simulink model "smartCart5_1work"  (R2016a)
settings: Solver=FixedStepDiscrete  StartTime=0.0  StopTime=inf  FixedStep=1  RelTol=1e-3
libraries: simulink x213, hdlsllib x84
(part 2 of 4)

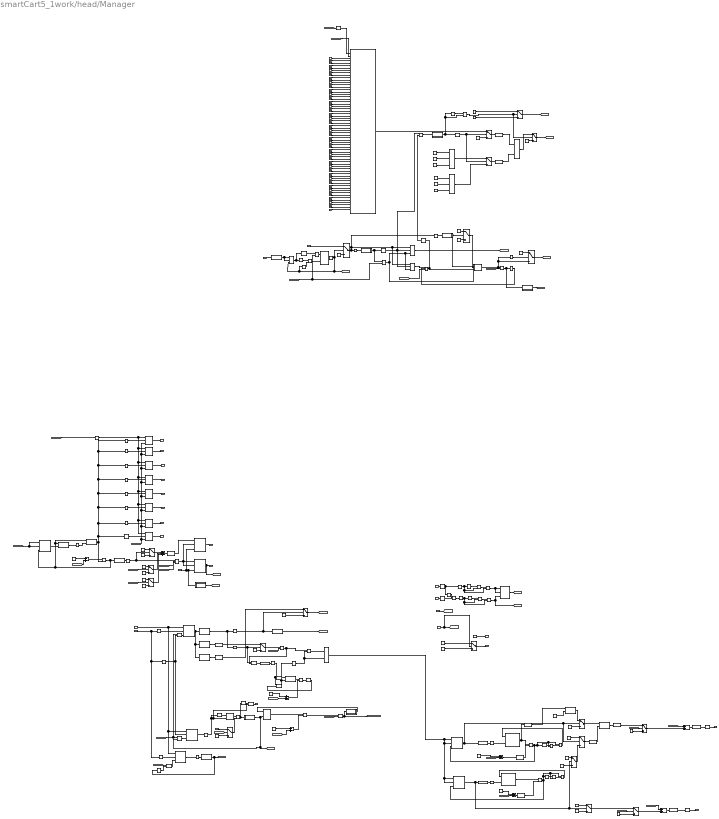
== system smartCart5_1work/head/Manager ==
  note: Декодер команд
  note: Схема декодирования команд
  note: Схема синхр
  note: Схема включения и выключения
  note: Схема управления приёмника
  note: Схема управления передатчиком
  AdrrIN : Inport  OutDataTypeStr=uint8
  DataIN : Inport  Port=2  OutDataTypeStr=uint32
  Start : Inport  Port=3  OutDataTypeStr=boolean
  Stop : Inport  Port=4  OutDataTypeStr=boolean
  RD : Inport  Port=5  OutDataTypeStr=boolean
  STEP : Inport  Port=6  OutDataTypeStr=uint8
  RST_IRQ : Inport  Port=7  OutDataTypeStr=boolean
  Number_write_byte : Inport  Port=8  OutDataTypeStr=uint8
  ON_TRANSMITE : Inport  Port=9  OutDataTypeStr=boolean
  time_pause : Inport  Port=10  OutDataTypeStr=uint32
  data_in_0 : Inport  Port=11  OutDataTypeStr=uint32
  data_in_1 : Inport  Port=12  OutDataTypeStr=uint32
  data_in_2 : Inport  Port=13  OutDataTypeStr=uint32
  data_in_3 : Inport  Port=14  OutDataTypeStr=uint32
  data_in_4 : Inport  Port=15  OutDataTypeStr=uint32
  data_in_5 : Inport  Port=16  OutDataTypeStr=uint32
  data_in_6 : Inport  Port=17  OutDataTypeStr=uint32
  data_in_7 : Inport  Port=18  OutDataTypeStr=uint32
  data_in_8 : Inport  Port=19  OutDataTypeStr=uint32
  data_in_9 : Inport  Port=20  OutDataTypeStr=uint32
  data_in_10 : Inport  Port=21  OutDataTypeStr=uint32
  data_in_11 : Inport  Port=22  OutDataTypeStr=uint32
  data_in_12 : Inport  Port=23  OutDataTypeStr=uint32
  data_in_13 : Inport  Port=24  OutDataTypeStr=uint32
  data_in_14 : Inport  Port=25  OutDataTypeStr=uint32
  data_in_15 : Inport  Port=26  OutDataTypeStr=uint32
  data_in_16 : Inport  Port=27  OutDataTypeStr=uint32
  data_in_17 : Inport  Port=28  OutDataTypeStr=uint32
  data_in_18 : Inport  Port=29  OutDataTypeStr=uint32
  data_in_19 : Inport  Port=30  OutDataTypeStr=uint32
  data_in_20 : Inport  Port=31  OutDataTypeStr=uint32
  data_in_21 : Inport  Port=32  OutDataTypeStr=uint32
  data_in_22 : Inport  Port=33  OutDataTypeStr=uint32
  data_in_23 : Inport  Port=34  OutDataTypeStr=uint32
  data_in_24 : Inport  Port=35  OutDataTypeStr=uint32
  data_in_25 : Inport  Port=36  OutDataTypeStr=uint32
  data_in_26 : Inport  Port=37  OutDataTypeStr=uint32
  data_in_27 : Inport  Port=38  OutDataTypeStr=uint32
  data_in_28 : Inport  Port=39  OutDataTypeStr=uint32
  data_in_29 : Inport  Port=40  OutDataTypeStr=uint32
  data_in_30 : Inport  Port=41  OutDataTypeStr=uint32
  data_in_31 : Inport  Port=42  OutDataTypeStr=uint32
  data_in_32 : Inport  Port=43  OutDataTypeStr=uint32
  data_in_33 : Inport  Port=44  OutDataTypeStr=uint32
  data_in_34 : Inport  Port=45  OutDataTypeStr=uint32
  data_in_35 : Inport  Port=46  OutDataTypeStr=uint32
  data_in_36 : Inport  Port=47  OutDataTypeStr=uint32
  data_in_37 : Inport  Port=48  OutDataTypeStr=uint32
  data_in_38 : Inport  Port=49  OutDataTypeStr=uint32
  data_in_39 : Inport  Port=50  OutDataTypeStr=uint32
  data_in_40 : Inport  Port=51  OutDataTypeStr=uint32
  data_in_41 : Inport  Port=52  OutDataTypeStr=uint32
  data_in_42 : Inport  Port=53  OutDataTypeStr=uint32
  data_in_43 : Inport  Port=54  OutDataTypeStr=uint32
  data_in_44 : Inport  Port=55  OutDataTypeStr=uint32
  data_in_45 : Inport  Port=56  OutDataTypeStr=uint32
  data_in_46 : Inport  Port=57  OutDataTypeStr=uint32
  data_in_47 : Inport  Port=58  OutDataTypeStr=uint32
  data_in_48 : Inport  Port=59  OutDataTypeStr=uint32
  data_in_49 : Inport  Port=60  OutDataTypeStr=uint32
  data_in_50 : Inport  Port=61  OutDataTypeStr=uint32
  data_in_51 : Inport  Port=62  OutDataTypeStr=uint32
  data_in_52 : Inport  Port=63  OutDataTypeStr=uint32
  data_in_53 : Inport  Port=64  OutDataTypeStr=uint32
  data_in_54 : Inport  Port=65  OutDataTypeStr=uint32
  data_in_55 : Inport  Port=66  OutDataTypeStr=uint32
  data_in_56 : Inport  Port=67  OutDataTypeStr=uint32
  data_in_57 : Inport  Port=68  OutDataTypeStr=uint32
  data_in_58 : Inport  Port=69  OutDataTypeStr=uint32
  data_in_59 : Inport  Port=70  OutDataTypeStr=uint32
  data_in_60 : Inport  Port=71  OutDataTypeStr=uint32
  data_in_61 : Inport  Port=72  OutDataTypeStr=uint32
  data_in_62 : Inport  Port=73  OutDataTypeStr=uint32
  data_in_63 : Inport  Port=74  OutDataTypeStr=uint32
  Add{,1..5,7} (7 alike) : Sum
  Add6 : Sum  Inputs=+++
  Atomic Subsystem : Subsystem  TreatAsAtomicUnit=on
  Bit Concat : hdlsllib/HDL Operations/Bit Concat  numInputs=2
  Bit Concat1 : hdlsllib/HDL Operations/Bit Concat  numInputs=2
  Bit Concat2 : hdlsllib/HDL Operations/Bit Concat  numInputs=3
  Bit Concat3 : hdlsllib/HDL Operations/Bit Concat  numInputs=3
  Bit Concat4 : hdlsllib/HDL Operations/Bit Concat  numInputs=2
  Bit Slice3 : hdlsllib/HDL Operations/Bit Slice  lidx=1  ridx=0
  Bit Slice4 : hdlsllib/HDL Operations/Bit Slice  lidx=9  ridx=2
  Bit Slice5 : hdlsllib/HDL Operations/Bit Slice  lidx=17  ridx=10
  Compare To Constant{,1..6,10,12,22,26} (11 alike) : simulink/Logic and Bit Operations/Compare To Constant  relop===  const=1  OutDataTypeStr=boolean
  Compare To Constant11 : simulink/Logic and Bit Operations/Compare To Constant  relop===  const=4  OutDataTypeStr=boolean
  Compare To Constant13 : simulink/Logic and Bit Operations/Compare To Constant  relop===  const=2  OutDataTypeStr=boolean
  Compare To Constant14 : simulink/Logic and Bit Operations/Compare To Constant  relop===  const=5  OutDataTypeStr=boolean
  Compare To Constant15 : simulink/Logic and Bit Operations/Compare To Constant  relop===  const=6  OutDataTypeStr=boolean
  Compare To Constant16 : simulink/Logic and Bit Operations/Compare To Constant  relop===  const=7  OutDataTypeStr=boolean
  Compare To Constant17 : simulink/Logic and Bit Operations/Compare To Constant  relop===  const=8  OutDataTypeStr=boolean
  Compare To Constant18 : simulink/Logic and Bit Operations/Compare To Constant  relop=~=  const=255  OutDataTypeStr=boolean
  Compare To Constant19 : simulink/Logic and Bit Operations/Compare To Constant  relop===  const=100  OutDataTypeStr=boolean
  Compare To Constant23 : simulink/Logic and Bit Operations/Compare To Constant  relop===  const=255  OutDataTypeStr=boolean
  Compare To Constant24 : simulink/Logic and Bit Operations/Compare To Constant  relop===  const=0  OutDataTypeStr=boolean
  Compare To Constant25 : simulink/Logic and Bit Operations/Compare To Constant  relop===  const=6  OutDataTypeStr=boolean
  Compare To Constant7 : simulink/Logic and Bit Operations/Compare To Constant  relop===  const=2  OutDataTypeStr=boolean
  Compare To Constant8 : simulink/Logic and Bit Operations/Compare To Constant  relop===  const=3  OutDataTypeStr=boolean
  Compare To Constant9 : simulink/Logic and Bit Operations/Compare To Constant  relop===  const=2  OutDataTypeStr=boolean
  Constant{,2,12..15,23,25,28,36} (10 alike) : Constant  Value=0  OutDataTypeStr=uint8  SampleTime=-1
  Constant{1,3,7,10,24} (5 alike) : Constant  OutDataTypeStr=uint8  SampleTime=-1
  Constant11 : Constant  Value=4  OutDataTypeStr=uint8  SampleTime=-1
  Constant{5,16,18,26} (4 alike) : Constant  OutDataTypeStr=boolean  SampleTime=-1
  Constant{6,17,22,31,33..34,38} (7 alike) : Constant  Value=0  OutDataTypeStr=uint32  SampleTime=-1
  Constant19 : Constant  Value=0  OutDataTypeStr=boolean  SampleTime=-1
  Constant20 : Constant  Value=0  OutDataTypeStr=boolean  SampleTime=-1
  Constant21 : Constant  Value=0  OutDataTypeStr=boolean  SampleTime=-1
  Constant27 : Constant  Value=2  OutDataTypeStr=uint8  SampleTime=-1
  Constant29 : Constant  Value=255  OutDataTypeStr=uint8  SampleTime=-1
  Constant30 : Constant  OutDataTypeStr=uint32  SampleTime=-1
  Constant32 : Constant  Value=2  OutDataTypeStr=uint32  SampleTime=-1
  Constant35 : Constant  Value=255  OutDataTypeStr=uint8  SampleTime=-1
  Constant37 : Constant  Value=3  OutDataTypeStr=uint32  SampleTime=-1
  Constant4 : Constant  Value=2  OutDataTypeStr=uint8  SampleTime=-1
  Constant40 : Constant  OutDataTypeStr=uint32  SampleTime=-1
  Constant8 : Constant  OutDataTypeStr=uint32  SampleTime=-1
  Constant9 : Constant  Value=2  OutDataTypeStr=uint8  SampleTime=-1
  Data Type Conversion{,3..4,7..8} (5 alike) : DataTypeConversion  OutDataTypeStr=uint8
  Data Type Conversion1 : DataTypeConversion  OutDataTypeStr=uint32
  Data Type Conversion10 : DataTypeConversion  OutDataTypeStr=fixdt(0,2,0)
  Data Type Conversion11 : DataTypeConversion  OutDataTypeStr=fixdt(0,3,0)
  Data Type Conversion12 : DataTypeConversion  OutDataTypeStr=uint32
  Data Type Conversion5 : DataTypeConversion  OutDataTypeStr=uint32
  Data Type Conversion6 : DataTypeConversion  OutDataTypeStr=fixdt(0,4,0)
  Data Type Conversion9 : DataTypeConversion  OutDataTypeStr=fixdt(0,4,0)
  Delay{,1..3,5..17} (17 alike) : Delay  DelayLength=1  InitialCondition=0
  Delay4 : Delay  DelayLength=3  InitialCondition=0
  HDL Counter1 : hdlsllib/HDL Operations/HDL Counter  CountType=Free running  CountInit=0  CountStep=1  CountMax=25  CountFromType=Initial value  CountFrom=0  CountResetPort=on  CountLoadPort=off  CountEnbPort=on  CountDirPort=off  CountDataType=Unsigned  CountWordLen=4  CountFracLen=0  CountSampTime=1
  HDL Counter10 : hdlsllib/HDL Operations/HDL Counter  CountType=Free running  CountInit=255  CountStep=1  CountMax=25  CountFromType=Initial value  CountFrom=255  CountResetPort=on  CountLoadPort=off  CountEnbPort=on  CountDirPort=off  CountDataType=Unsigned  CountWordLen=8  CountFracLen=0  CountSampTime=1
  HDL Counter12 : hdlsllib/HDL Operations/HDL Counter  CountType=Count limited  CountInit=0  CountStep=1  CountMax=100  CountFromType=Initial value  CountFrom=0  CountResetPort=on  CountLoadPort=off  CountEnbPort=on  CountDirPort=off  CountDataType=Unsigned  CountWordLen=8  CountFracLen=0  CountSampTime=1
  HDL Counter13 : hdlsllib/HDL Operations/HDL Counter  CountType=Free running  CountInit=0  CountStep=1  CountMax=5208*2  CountFromType=Initial value  CountFrom=0  CountResetPort=on  CountLoadPort=off  CountEnbPort=on  CountDirPort=off  CountDataType=Unsigned  CountWordLen=32  CountFracLen=0  CountSampTime=1
  HDL Counter2 : hdlsllib/HDL Operations/HDL Counter  CountType=Free running  CountInit=0  CountStep=1  CountMax=25  CountFromType=Initial value  CountFrom=0  CountResetPort=on  CountLoadPort=off  CountEnbPort=on  CountDirPort=off  CountDataType=Unsigned  CountWordLen=4  CountFracLen=0  CountSampTime=1
  HDL Counter3 : hdlsllib/HDL Operations/HDL Counter  CountType=Free running  CountInit=0  CountStep=1  CountMax=25  CountFromType=Initial value  CountFrom=0  CountResetPort=on  CountLoadPort=off  CountEnbPort=on  CountDirPort=off  CountDataType=Unsigned  CountWordLen=8  CountFracLen=0  CountSampTime=1
  HDL Counter4 : hdlsllib/HDL Operations/HDL Counter  CountType=Free running  CountInit=0  CountStep=1  CountMax=25  CountFromType=Initial value  CountFrom=0  CountResetPort=on  CountLoadPort=off  CountEnbPort=on  CountDirPort=off  CountDataType=Unsigned  CountWordLen=4  CountFracLen=0  CountSampTime=1
  HDL Counter5 : hdlsllib/HDL Operations/HDL Counter  CountType=Free running  CountInit=0  CountStep=1  CountMax=25  CountFromType=Initial value  CountFrom=0  CountResetPort=off  CountLoadPort=off  CountEnbPort=on  CountDirPort=off  CountDataType=Unsigned  CountWordLen=1  CountFracLen=0  CountSampTime=1
  HDL Counter6 : hdlsllib/HDL Operations/HDL Counter  CountType=Free running  CountInit=0  CountStep=1  CountMax=25  CountFromType=Initial value  CountFrom=0  CountResetPort=off  CountLoadPort=off  CountEnbPort=on  CountDirPort=off  CountDataType=Unsigned  CountWordLen=1  CountFracLen=0  CountSampTime=1
  HDL Counter7 : hdlsllib/HDL Operations/HDL Counter  CountType=Free running  CountInit=0  CountStep=1  CountMax=25  CountFromType=Initial value  CountFrom=0  CountResetPort=off  CountLoadPort=off  CountEnbPort=on  CountDirPort=off  CountDataType=Unsigned  CountWordLen=1  CountFracLen=0  CountSampTime=1
  HDL Counter8 : hdlsllib/HDL Operations/HDL Counter  CountType=Free running  CountInit=0  CountStep=1  CountMax=25  CountFromType=Initial value  CountFrom=0  CountResetPort=on  CountLoadPort=off  CountEnbPort=on  CountDirPort=off  CountDataType=Unsigned  CountWordLen=1  CountFracLen=0  CountSampTime=1
  HDL Counter9 : hdlsllib/HDL Operations/HDL Counter  CountType=Free running  CountInit=0  CountStep=1  CountMax=25  CountFromType=Initial value  CountFrom=0  CountResetPort=on  CountLoadPort=on  CountEnbPort=on  CountDirPort=off  CountDataType=Unsigned  CountWordLen=8  CountFracLen=0  CountSampTime=1
  Logical Operator{,2,7,10} (4 alike) : Logic  Operator=XOR  AllPortsSameDT=off  OutDataTypeStr=boolean
  Logical Operator{1,3..4,6,8..9,12,15,17,19,26,32} (12 alike) : Logic  AllPortsSameDT=off  OutDataTypeStr=boolean
  Logical Operator{5,11,16,18,25,31} (6 alike) : Logic  Operator=NOT  AllPortsSameDT=off  OutDataTypeStr=boolean
  Logical Operator{13..14,20,22,24,28,30} (7 alike) : Logic  Operator=OR  AllPortsSameDT=off  OutDataTypeStr=boolean
  Logical Operator23 : Logic  Operator=OR  Inputs=3  AllPortsSameDT=off  OutDataTypeStr=boolean
  Logical Operator27 : Logic  Inputs=3  AllPortsSameDT=off  OutDataTypeStr=boolean
  Logical Operator29 : Logic  Operator=NOT  Inputs=3  AllPortsSameDT=off  OutDataTypeStr=boolean
  Relational Operator{,1..4,6..8} (8 alike) : RelationalOperator  Operator===  OutDataTypeStr=boolean
  Switch{1..19,21} (20 alike) : Switch  Criteria=u2 ~= 0
  Unit Delay Enabled Resettable{,1..2,5..13,15,25} (14 alike) : simulink/Additional Math & Discrete/Additional Discrete/Unit Delay Enabled Resettable  vinit=0.0  tsamp=-1
  Unit Delay Enabled Resettable{3..4,14,16,26,28} (6 alike) : simulink/Additional Math & Discrete/Additional Discrete/Unit Delay Enabled Resettable  vinit=0  tsamp=-1
  signal_edg : Subsystem  TreatAsAtomicUnit=on
  signal_edg1 : Subsystem  TreatAsAtomicUnit=on
  signal_edg10 : Subsystem  TreatAsAtomicUnit=on
  signal_edg11 : Subsystem  TreatAsAtomicUnit=on
  signal_edg12 : Subsystem  TreatAsAtomicUnit=on
  signal_edg2 : Subsystem  TreatAsAtomicUnit=on
  signal_edg3 : Subsystem  TreatAsAtomicUnit=on
  signal_edg4 : Subsystem  TreatAsAtomicUnit=on
  signal_edg6 : Subsystem  TreatAsAtomicUnit=on
  signal_edg7 : Subsystem  TreatAsAtomicUnit=on
  signal_edg8 : Subsystem  TreatAsAtomicUnit=on
  signal_edg9 : Subsystem  TreatAsAtomicUnit=on
  addrout : Outport  OutDataTypeStr=uint8
  DATA_OUT : Outport  Port=2  OutDataTypeStr=uint32
  Out1 : Outport  Port=3  OutDataTypeStr=uint8
  Out2 : Outport  Port=4  OutDataTypeStr=uint8
  Out3 : Outport  Port=5  OutDataTypeStr=uint8
  Out4 : Outport  Port=6  OutDataTypeStr=uint8
  Out5 : Outport  Port=7  OutDataTypeStr=uint8
  Out6 : Outport  Port=8  OutDataTypeStr=uint8
  Out7 : Outport  Port=9  OutDataTypeStr=uint8
  Out8 : Outport  Port=10  OutDataTypeStr=uint8
  irq : Outport  Port=11  OutDataTypeStr=boolean
  addr_mux : Outport  Port=12  OutDataTypeStr=uint8
  data_mux : Outport  Port=13  OutDataTypeStr=uint32
  STATUS : Outport  Port=14  OutDataTypeStr=uint32
  rd_switch : Outport  Port=15  OutDataTypeStr=boolean
  wires:
  Compare To Constant/1 -> Logical Operator1/2, Logical Operator/2, Delay/1
  Delay/1 -> Logical Operator/1
  Logical Operator/1 -> Logical Operator1/1
  Logical Operator1/1 -> Unit Delay Enabled Resettable/2, Unit Delay Enabled Resettable/1
  Compare To Constant1/1 -> Logical Operator3/2, Logical Operator2/2, Delay1/1
  Delay1/1 -> Logical Operator2/1
  Logical Operator2/1 -> Logical Operator3/1
  Logical Operator5/1 -> Logical Operator4/1
  Logical Operator4/1 -> Compare To Constant1/1
  Logical Operator3/1 -> Unit Delay Enabled Resettable/3, [RST]
  Unit Delay Enabled Resettable/1 -> [EN]
  HDL Counter2/1 -> Relational Operator2/1
  Bit Slice4/1 -> Data Type Conversion7/1
  Bit Slice5/1 -> Data Type Conversion8/1
  Bit Slice3/1 -> Compare To Constant10/1, Compare To Constant9/1
  Data Type Conversion8/1 -> Switch9/1
  Constant14/1 -> Switch9/3
  Data Type Conversion7/1 -> Switch10/1
  Constant15/1 -> Switch10/3
  Unit Delay Enabled Resettable1/1 -> Bit Slice5/1, Bit Slice4/1, Bit Slice3/1
  AdrrIN/1 -> Compare To Constant25/1, Compare To Constant13/1, Compare To Constant12/1
  Compare To Constant12/1 -> Unit Delay Enabled Resettable1/2
  HDL Counter1/1 -> Relational Operator1/1, Data Type Conversion/1
  Constant1/1 -> Switch1/1
  Constant2/1 -> Switch1/3
  Switch2/1 -> Bit Concat/1
  Constant/1 -> Switch2/3
  Constant4/1 -> Switch3/1
  Data Type Conversion/1 -> Bit Concat1/1
  Constant5/1 -> Bit Concat1/2
  Bit Concat1/1 -> Switch2/1
  Bit Concat/1 -> Data Type Conversion1/1
  Switch10/1 -> Relational Operator/1
  STEP/1 -> [INST_WORK_VAL]
  [INST_WORK_VAL] -> Relational Operator/2
  [INST_WORK_VAL] -> Add/2
  Constant9/1 -> Add/1
  Logical Operator8/1 -> Unit Delay Enabled Resettable4/2, Unit Delay Enabled Resettable4/1, Unit Delay Enabled Resettable3/2, Unit Delay Enabled Resettable3/1
  Data Type Conversion1/1 -> Switch12/1
  Constant22/1 -> Switch12/3
  [INST_WORK] -> Switch12/2
  Switch1/1 -> Switch13/1
  [INST_WORK] -> Switch13/2
  Constant23/1 -> Switch13/3
  Switch12/1 -> Add2/2
  Switch13/1 -> Add1/2
  Add1/1 -> Data Type Conversion4/1
  Add2/1 -> Data Type Conversion5/1
  Delay6/1 -> Logical Operator17/2, Logical Operator8/2
  Add/1 -> Data Type Conversion6/1
  Data Type Conversion6/1 -> Relational Operator2/2
  [INST_WORK_VAL] -> Add3/2
  Constant24/1 -> Add3/1
  Add3/1 -> Data Type Conversion9/1
  Data Type Conversion9/1 -> Relational Operator1/2
  Delay7/1 -> DATA_OUT/1
  Data Type Conversion5/1 -> Delay7/1
  Delay8/1 -> addrout/1
  Data Type Conversion4/1 -> Delay8/1
  Constant3/1 -> Switch14/1
  Switch3/1 -> Data Type Conversion10/1
  Data Type Conversion10/1 -> Bit Concat/2
  Switch14/1 -> Switch3/3
  Constant25/1 -> Switch14/3
  Logical Operator17/1 -> Logical Operator8/1
  Relational Operator/1 -> Logical Operator19/2, Logical Operator17/1
  Unit Delay Enabled Resettable3/1 -> HDL Counter6/1, Switch3/2, Switch2/2
  Unit Delay Enabled Resettable4/1 -> Switch14/2, Switch1/2, HDL Counter7/1
  [addr_wr] -> Add1/1
  [data_wr] -> Add2/1
  Logical Operator7/1 -> Logical Operator6/2
  Delay2/1 -> Logical Operator7/1
  Relational Operator1/1 -> Unit Delay Enabled Resettable3/3, Logical Operator6/1, Logical Operator7/2, Delay2/1
  Logical Operator6/1 -> HDL Counter1/1
  Logical Operator10/1 -> Logical Operator9/2
  Delay3/1 -> Logical Operator10/1
  Relational Operator2/1 -> Unit Delay Enabled Resettable4/3, Delay3/1, Logical Operator9/1, Logical Operator10/2
  Logical Operator9/1 -> HDL Counter2/1
  Compare To Constant10/1 -> Logical Operator19/1, Switch10/2
  Logical Operator11/1 -> HDL Counter4/1
  HDL Counter4/1 -> Relational Operator4/1
  [INST_WORK_VAL] -> Add5/2
  Add5/1 -> Relational Operator4/2
  Constant10/1 -> Add5/1
  Logical Operator12/1 -> Delay6/1, HDL Counter4/2
  Relational Operator4/1 -> Logical Operator18/1
  Logical Operator18/1 -> Logical Operator12/2
  HDL Counter5/1 -> Compare To Constant3/1
  Logical Operator19/1 -> HDL Counter5/1
  Compare To Constant3/1 -> Logical Operator12/1, Logical Operator11/1
  HDL Counter6/1 -> Compare To Constant4/1
  Compare To Constant4/1 -> HDL Counter1/2
  HDL Counter7/1 -> Compare To Constant5/1
  Compare To Constant5/1 -> HDL Counter2/2
  Compare To Constant9/1 -> Switch9/2, signal_edg/1(In1)
  Switch9/1 -> [RD_BYTE_VAL]
  RD/1 -> Switch5/2, [INST_WORK]
  Logical Operator13/1 -> Unit Delay Enabled Resettable2/3
  [RST] -> Logical Operator14/1, Logical Operator13/1
  Logical Operator14/1 -> Unit Delay Enabled Resettable1/3
  signal_edg/1(Out1) -> [RD_BYTE]
  [RD_BYTE] -> Unit Delay Enabled Resettable5/1, Unit Delay Enabled Resettable5/2
  Unit Delay Enabled Resettable5/1 -> HDL Counter8/2
  HDL Counter8/1 -> Compare To Constant2/1
  Compare To Constant2/1 -> HDL Counter3/2
  Constant7/1 -> Add4/1
  Add4/1 -> Relational Operator3/1
  [INST_WORK_VAL] -> Add4/2
  Relational Operator3/1 -> signal_edg4/1(In1), Unit Delay Enabled Resettable5/3, HDL Counter8/1, HDL Counter3/1
  Compare To Constant6/1 -> Unit Delay Enabled Resettable6/2
  Compare To Constant7/1 -> Unit Delay Enabled Resettable7/2
  Compare To Constant8/1 -> Unit Delay Enabled Resettable8/2
  Compare To Constant11/1 -> Unit Delay Enabled Resettable9/2
  Compare To Constant14/1 -> Unit Delay Enabled Resettable10/2
  Compare To Constant15/1 -> Unit Delay Enabled Resettable11/2
  Compare To Constant16/1 -> Unit Delay Enabled Resettable12/2
  Compare To Constant17/1 -> Unit Delay Enabled Resettable13/2
  HDL Counter3/1 -> Compare To Constant17/1, Compare To Constant16/1, Compare To Constant14/1, Compare To Constant11/1, Compare To Constant8/1, Compare To Constant6/1, Compare To Constant7/1, Compare To Constant15/1, Relational Operator3/2
  Unit Delay Enabled Resettable6/1 -> Out1/1
  Unit Delay Enabled Resettable7/1 -> Out2/1
  Unit Delay Enabled Resettable8/1 -> Out3/1
  Unit Delay Enabled Resettable9/1 -> Out4/1
  Unit Delay Enabled Resettable10/1 -> Out5/1
  Unit Delay Enabled Resettable11/1 -> Out6/1
  Unit Delay Enabled Resettable12/1 -> Out7/1
  Unit Delay Enabled Resettable13/1 -> Out8/1
  [RST] -> Unit Delay Enabled Resettable9/3, Unit Delay Enabled Resettable8/3, Unit Delay Enabled Resettable7/3, Unit Delay Enabled Resettable6/3, Unit Delay Enabled Resettable10/3, Unit Delay Enabled Resettable11/3, Unit Delay Enabled Resettable12/3, Unit Delay Enabled Resettable13/3
  Delay4/1 -> Unit Delay Enabled Resettable9/1, Unit Delay Enabled Resettable12/1, Unit Delay Enabled Resettable13/1, Unit Delay Enabled Resettable11/1, Unit Delay Enabled Resettable10/1, Unit Delay Enabled Resettable8/1, Unit Delay Enabled Resettable7/1, Unit Delay Enabled Resettable6/1
  Unit Delay Enabled Resettable14/1 -> [interrypt], irq/1
  RST_IRQ/1 -> Unit Delay Enabled Resettable26/3, signal_edg10/1(In1), Unit Delay Enabled Resettable14/3
  Constant6/1 -> Switch5/1
  Constant8/1 -> Switch5/3
  Switch5/1 -> data_mux/1
  Constant11/1 -> addr_mux/1
  [RD_BYTE_VAL] -> Delay4/1
  ? -> ?
  Atomic Subsystem/1(DataOut) -> Switch6/1
  Constant17/1 -> Switch6/3
  Constant16/1 -> Bit Concat2/3
  Constant18/1 -> Bit Concat2/2
  Constant19/1 -> Bit Concat2/1
  Constant20/1 -> Bit Concat3/3
  Constant21/1 -> Bit Concat3/2
  Constant26/1 -> Bit Concat3/1
  Bit Concat2/1 -> Switch7/1
  Bit Concat3/1 -> Switch7/3
  Switch6/1 -> Data Type Conversion3/1
  Switch7/1 -> Data Type Conversion11/1
  Data Type Conversion3/1 -> Bit Concat4/1
  Data Type Conversion11/1 -> Bit Concat4/2
  signal_edg2/1(Out1) -> Delay11/1, Logical Operator22/2, Delay10/1
  Delay10/1 -> Switch7/2, Switch6/2
  Delay11/1 -> Logical Operator22/1
  Logical Operator22/1 -> Switch16/2, Switch8/2
  Constant27/1 -> Switch8/1
  Constant28/1 -> Switch8/3
  Bit Concat4/1 -> Switch16/1
  [count_wr] -> Delay12/1
  Unit Delay Enabled Resettable26/1 -> STATUS/1
  Delay5/1 -> Switch11/2, Logical Operator23/1
  Logical Operator23/1 -> Unit Delay Enabled Resettable26/2, Unit Delay Enabled Resettable14/1, Unit Delay Enabled Resettable14/2
  Constant30/1 -> Switch11/1
  Constant31/1 -> Switch11/3
  Switch11/1 -> Add6/1
  Switch15/1 -> Add6/2
  Constant32/1 -> Switch15/1
  Constant33/1 -> Switch15/3
  [IRQ_TRANSMIT] -> Switch15/2
  [IRQ_TRANSMIT] -> Logical Operator23/2
  signal_edg4/1(Out1) -> Delay5/1
  Add6/1 -> Data Type Conversion12/1
  Data Type Conversion12/1 -> Unit Delay Enabled Resettable26/1
  HDL Counter10/1 -> Relational Operator7/1
  signal_edg12/1(Out1) -> Logical Operator13/2, [byte_done], HDL Counter10/2
  Start/1 -> Delay13/1
  Delay13/1 -> Logical Operator5/1, Compare To Constant/1
  Stop/1 -> Delay14/1
  Delay14/1 -> Logical Operator4/2
  Constant34/1 -> Switch16/3
  Switch16/1 -> [data_wr]
  Switch8/1 -> [addr_wr]
  Constant35/1 -> Switch17/3
  Unit Delay Enabled Resettable15/1 -> [num_wr_byt]
  [ON_TRANS] -> Logical Operator26/2
  Compare To Constant18/1 -> signal_edg1/1(In1)
  Relational Operator7/1 -> Logical Operator26/1
  Number_write_byte/1 -> Switch17/1
  Switch17/1 -> Compare To Constant24/1, Unit Delay Enabled Resettable28/1, Unit Delay Enabled Resettable15/1, Compare To Constant18/1
  HDL Counter9/1 -> Switch4/3, Compare To Constant23/1, Relational Operator8/1
  [num_wr_byt] -> Relational Operator8/2
  Unit Delay Enabled Resettable28/1 -> Logical Operator27/1
  Logical Operator27/1 -> Delay15/1, HDL Counter9/4
  Relational Operator8/1 -> signal_edg6/1(In1), Logical Operator29/1
  Logical Operator29/1 -> Logical Operator27/2
  Delay9/1 -> Unit Delay Enabled Resettable15/2, Unit Delay Enabled Resettable28/2, Logical Operator28/1
  signal_edg1/1(Out1) -> Logical Operator20/1, Delay9/1
  Logical Operator28/1 -> signal_edg2/1(In1)
  [byte_done] -> Logical Operator27/3
  Delay15/1 -> Logical Operator28/2
  signal_edg6/1(Out1) -> [write_ok]
  [num_wr_byt] -> Add7/2
  Add7/1 -> Relational Operator7/2
  Constant12/1 -> Add7/1
  Logical Operator26/1 -> signal_edg3/1(In1), [IRQ_TRANSMIT]
  ON_TRANSMITE/1 -> signal_edg7/1(In1)
  signal_edg7/1(Out1) -> Unit Delay Enabled Resettable16/2, Unit Delay Enabled Resettable16/1
  HDL Counter12/1 -> Compare To Constant19/1
  Compare To Constant19/1 -> Switch17/2, Logical Operator16/1, Unit Delay Enabled Resettable16/3, [ON_TRANS]
  signal_edg3/1(Out1) -> HDL Counter10/1
  Unit Delay Enabled Resettable16/1 -> signal_edg8/1(In1), Delay16/1
  Delay16/1 -> Logical Operator15/1
  Logical Operator15/1 -> HDL Counter12/2
  Logical Operator16/1 -> Logical Operator15/2
  Compare To Constant23/1 -> Switch4/2
  Switch4/1 -> [count_wr]
  Constant13/1 -> Switch4/1
  Compare To Constant24/1 -> signal_edg9/1(In1)
  signal_edg9/1(Out1) -> HDL Counter9/2, Switch18/2
  Constant29/1 -> Switch18/1
  Constant36/1 -> Switch18/3
  Switch18/1 -> HDL Counter9/3
  signal_edg10/1(Out1) -> [rst_interrypt]
  Logical Operator20/1 -> HDL Counter9/1, Unit Delay Enabled Resettable28/3, Unit Delay Enabled Resettable15/3
  [rst_interrypt] -> Logical Operator24/2, Logical Operator20/2
  signal_edg8/1(Out1) -> Logical Operator24/1
  Logical Operator24/1 -> HDL Counter12/1
  Compare To Constant25/1 -> Unit Delay Enabled Resettable25/2
  Logical Operator30/1 -> Unit Delay Enabled Resettable25/3
  [RST] -> Logical Operator30/1
  Unit Delay Enabled Resettable25/1 -> Compare To Constant26/1
  Compare To Constant26/1 -> signal_edg11/1(In1)
  signal_edg11/1(Out1) -> Delay17/1, [interrypt_timer]
  Constant37/1 -> Switch19/1
  Constant38/1 -> Switch19/3
  Switch19/1 -> Add6/3
  [interrypt_timer] -> Switch19/2
  [interrypt_timer] -> Logical Operator23/3
  Delay17/1 -> Logical Operator30/2
  Compare To Constant13/1 -> Logical Operator14/2, Unit Delay Enabled Resettable2/2
  DataIN/1 -> Unit Delay Enabled Resettable25/1, Unit Delay Enabled Resettable2/1, Unit Delay Enabled Resettable1/1
  Unit Delay Enabled Resettable2/1 -> Compare To Constant22/1
  HDL Counter13/1 -> Relational Operator6/1
  Relational Operator6/1 -> Logical Operator25/1, signal_edg12/1(In1)
  Logical Operator31/1 -> HDL Counter13/1
  Compare To Constant22/1 -> Logical Operator31/1, Logical Operator32/2, HDL Counter13/2
  Constant40/1 -> Switch21/3
  Switch21/1 -> Relational Operator6/2
  [ON_TRANS] -> Switch21/2
  time_pause/1 -> Switch21/1
  Logical Operator25/1 -> Logical Operator32/1
  Logical Operator32/1 -> rd_switch/1
  [RST] -> Atomic Subsystem/2(rst)
  Delay12/1 -> Atomic Subsystem/1(addr)
  data_in_0/1 -> Atomic Subsystem/3(data_in_1)
  data_in_1/1 -> Atomic Subsystem/4(data_in_2)
  data_in_2/1 -> Atomic Subsystem/5(data_in_3)
  data_in_3/1 -> Atomic Subsystem/6(data_in_4)
  data_in_5/1 -> Atomic Subsystem/8(data_in_6)
  data_in_4/1 -> Atomic Subsystem/7(data_in_5)
  data_in_6/1 -> Atomic Subsystem/9(data_in_7)
  data_in_7/1 -> Atomic Subsystem/10(data_in_8)
  data_in_8/1 -> Atomic Subsystem/11(data_in_9)
  data_in_9/1 -> Atomic Subsystem/12(data_in_10)
  data_in_11/1 -> Atomic Subsystem/14(data_in_12)
  data_in_10/1 -> Atomic Subsystem/13(data_in_11)
  data_in_12/1 -> Atomic Subsystem/15(data_in_13)
  data_in_13/1 -> Atomic Subsystem/16(data_in_14)
  data_in_14/1 -> Atomic Subsystem/17(data_in_15)
  data_in_15/1 -> Atomic Subsystem/18(data_in_16)
  data_in_17/1 -> Atomic Subsystem/20(data_in_18)
  data_in_16/1 -> Atomic Subsystem/19(data_in_17)
  data_in_18/1 -> Atomic Subsystem/21(data_in_19)
  data_in_19/1 -> Atomic Subsystem/22(data_in_20)
  data_in_20/1 -> Atomic Subsystem/23(data_in_21)
  data_in_21/1 -> Atomic Subsystem/24(data_in_22)
  data_in_23/1 -> Atomic Subsystem/26(data_in_24)
  data_in_22/1 -> Atomic Subsystem/25(data_in_23)
  data_in_24/1 -> Atomic Subsystem/27(data_in_25)
  data_in_25/1 -> Atomic Subsystem/28(data_in_26)
  data_in_26/1 -> Atomic Subsystem/29(data_in_27)
  data_in_27/1 -> Atomic Subsystem/30(data_in_28)
  data_in_29/1 -> Atomic Subsystem/32(data_in_30)
  data_in_28/1 -> Atomic Subsystem/31(data_in_29)
  data_in_30/1 -> Atomic Subsystem/33(data_in_31)
  data_in_31/1 -> Atomic Subsystem/34(data_in_32)
  data_in_32/1 -> Atomic Subsystem/35(data_in_33)
  data_in_33/1 -> Atomic Subsystem/36(data_in_34)
  data_in_35/1 -> Atomic Subsystem/38(data_in_36)
  data_in_34/1 -> Atomic Subsystem/37(data_in_35)
  data_in_36/1 -> Atomic Subsystem/39(data_in_37)
  data_in_37/1 -> Atomic Subsystem/40(data_in_38)
  data_in_38/1 -> Atomic Subsystem/41(data_in_39)
  data_in_39/1 -> Atomic Subsystem/42(data_in_40)
  data_in_41/1 -> Atomic Subsystem/44(data_in_42)
  data_in_40/1 -> Atomic Subsystem/43(data_in_41)
  data_in_42/1 -> Atomic Subsystem/45(data_in_43)
  data_in_43/1 -> Atomic Subsystem/46(data_in_44)
  data_in_44/1 -> Atomic Subsystem/47(data_in_45)
  data_in_45/1 -> Atomic Subsystem/48(data_in_46)
  data_in_47/1 -> Atomic Subsystem/50(data_in_48)
  data_in_46/1 -> Atomic Subsystem/49(data_in_47)
  data_in_48/1 -> Atomic Subsystem/51(data_in_49)
  data_in_49/1 -> Atomic Subsystem/52(data_in_50)
  data_in_50/1 -> Atomic Subsystem/53(data_in_51)
  data_in_51/1 -> Atomic Subsystem/54(data_in_52)
  data_in_53/1 -> Atomic Subsystem/56(data_in_54)
  data_in_52/1 -> Atomic Subsystem/55(data_in_53)
  data_in_54/1 -> Atomic Subsystem/57(data_in_55)
  data_in_55/1 -> Atomic Subsystem/58(data_in_56)
  data_in_56/1 -> Atomic Subsystem/59(data_in_57)
  data_in_57/1 -> Atomic Subsystem/60(data_in_58)
  data_in_59/1 -> Atomic Subsystem/62(data_in_60)
  data_in_58/1 -> Atomic Subsystem/61(data_in_59)
  data_in_60/1 -> Atomic Subsystem/63(data_in_61)
  data_in_61/1 -> Atomic Subsystem/64(data_in_62)
  data_in_62/1 -> Atomic Subsystem/65(data_in_63)
  data_in_63/1 -> Atomic Subsystem/66(data_in_64)
